simulink model "hop_2D_sim"  (R2022b)
settings: Solver=FixedStepAuto  StartTime=0.0  StopTime=0.5  FixedStep=10e-4  RelTol=1e-3
values from neighbouring files (symbols this model uses):
  bl = 0.1    [twoD.m]
  g = 9.81    [twoD.m]
  k0 = 1000    [twoD.m]
  Kf = acker(Af,Bf,Poles)    [twoD.m]
  l0 = 0.3    [twoD.m]
  m = 0.5    [twoD.m]
  Nf = rscale(Gp,Kf)    [twoD.m]
undefined symbols (not defined in the file or in its folder): If, K, Kg, Ts
settings Model: Creator=phattanarat  LastModifiedBy=phattanarat

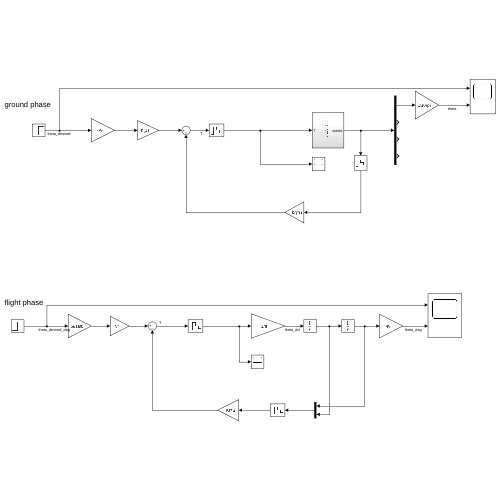
[thumbnail: Simulink's stored preview of the top-level diagram]
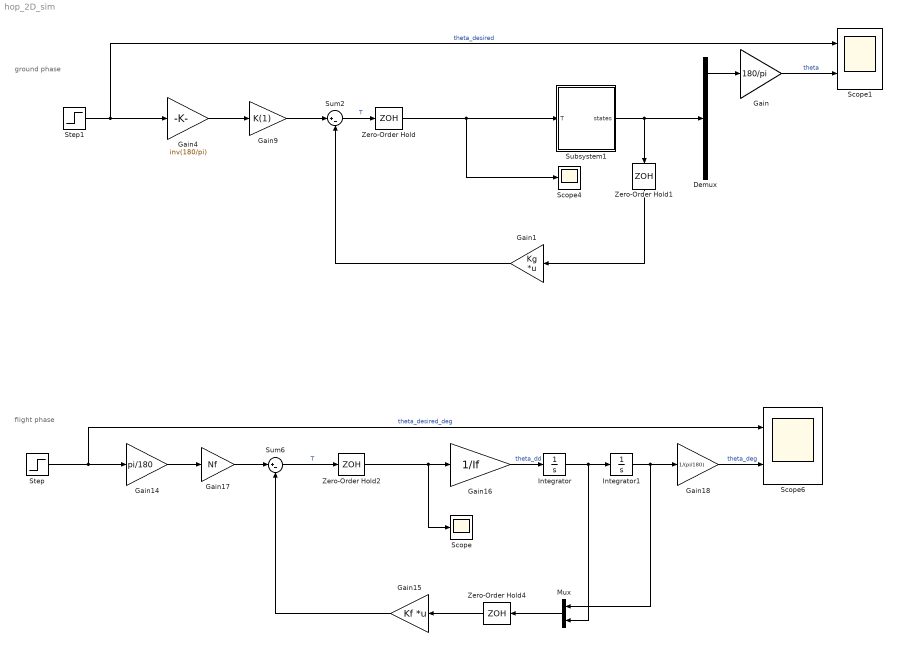
== system hop_2D_sim ==
  note: ground phase
  note: flight phase
  Demux : Demux
  Gain : Gain  Gain=180/pi
  Gain1 : Gain  Gain=Kg  Multiplication=Matrix(K*u)
  Gain14 : Gain  Gain=pi/180
  Gain15 : Gain  Gain=Kf  Multiplication=Matrix(K*u)
  Gain16 : Gain  Gain=1/If
  Gain17 : Gain  Gain=Nf
  Gain18 : Gain  Gain=1/(pi/180)
  Gain4 : Gain  Gain=inv(180/pi)
  Gain9 : Gain  Gain=K(1)
  Integrator : Integrator
  Integrator1 : Integrator  InitialCondition=deg2rad(95)
  Mux : Mux  Inputs=2
  Scope : Scope
  Scope1 : Scope  NumInputPorts=2
  Scope4 : Scope
  Scope6 : Scope  NumInputPorts=2
  Step : Step  Time=0  After=90  SampleTime=0
  Step1 : Step  Time=0  After=95  SampleTime=0
  Subsystem1 : Subsystem
  Sum2 : Sum  Inputs=|+-
  Sum6 : Sum  Inputs=|+-
  Zero-Order Hold{,1..2,4} (4 alike) : ZeroOrderHold  SampleTime=Ts
  wires:
  Gain9/1 -> Sum2/1
  Gain4/1 -> Gain9/1
  Sum2/1 -> Zero-Order Hold/1  "T"
  Step1/1 -> Scope1/1, Gain4/1  "theta_desired"
  Gain1/1 -> Sum2/2
  Gain14/1 -> Gain17/1
  Sum6/1 -> Zero-Order Hold2/1  "T"
  Gain16/1 -> Integrator/1  "theta_dd"
  Integrator1/1 -> Gain18/1, Mux/1
  Mux/1 -> Zero-Order Hold4/1
  Gain17/1 -> Sum6/1
  Gain18/1 -> Scope6/2  "theta_deg"
  Step/1 -> Scope6/1, Gain14/1  "theta_desired_deg"
  Subsystem1/1(states) -> Zero-Order Hold1/1, Demux/1
  Zero-Order Hold1/1 -> Gain1/1
  Demux/1 -> Gain/1
  Gain/1 -> Scope1/2  "theta"
  Integrator/1 -> Mux/2, Integrator1/1
  Zero-Order Hold4/1 -> Gain15/1
  Gain15/1 -> Sum6/2
  Zero-Order Hold/1 -> Scope4/1, Subsystem1/1(T)
  Zero-Order Hold2/1 -> Scope/1, Gain16/1

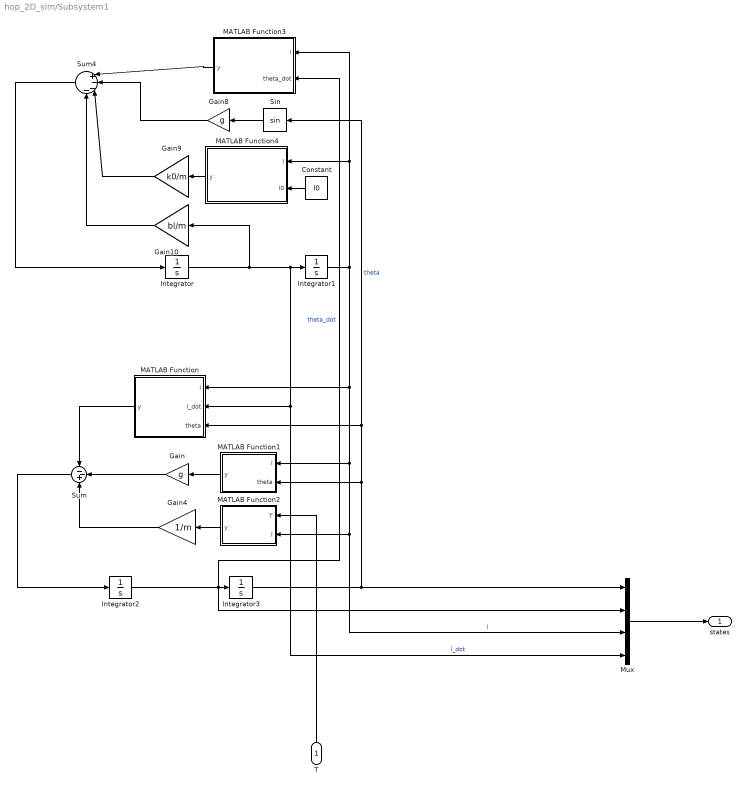
== system hop_2D_sim/Subsystem1 ==
  T : Inport
  Constant : Constant  Value=l0
  Gain : Gain  Gain=g
  Gain10 : Gain  Gain=bl/m
  Gain4 : Gain  Gain=1/m
  Gain8 : Gain  Gain=g
  Gain9 : Gain  Gain=k0/m
  Integrator : Integrator  InitialCondition=0.1
  Integrator1 : Integrator  InitialCondition=l0
  Integrator2 : Integrator
  Integrator3 : Integrator  InitialCondition=90*pi/180
  MATLAB Function : MATLAB Function  TreatAsAtomicUnit=on
  MATLAB Function1 : MATLAB Function  TreatAsAtomicUnit=on
  MATLAB Function2 : MATLAB Function  TreatAsAtomicUnit=on
  MATLAB Function3 : MATLAB Function  TreatAsAtomicUnit=on
  MATLAB Function4 : MATLAB Function  TreatAsAtomicUnit=on
  Mux : Mux
  Sin : Trigonometry
  Sum : Sum  Inputs=--+
  Sum4 : Sum  Inputs=|+---
  states : Outport
  wires:
  MATLAB Function4/1(y) -> Gain9/1
  MATLAB Function2/1(y) -> Gain4/1
  MATLAB Function1/1(y) -> Gain/1
  Integrator1/1 -> Mux/3, MATLAB Function2/2(l), MATLAB Function1/1(l), MATLAB Function/1(l), MATLAB Function4/1(l), MATLAB Function3/1(l)  "l"
  Integrator2/1 -> MATLAB Function3/2(theta_dot), Integrator3/1, Mux/2  "theta_dot"
  Sin/1 -> Gain8/1
  Integrator/1 -> Mux/4, MATLAB Function/2(l_dot), Integrator1/1, Gain10/1  "l_dot"
  Integrator3/1 -> MATLAB Function1/2(theta), MATLAB Function/3(theta), Sin/1, Mux/1  "theta"
  Constant/1 -> MATLAB Function4/2(l0)
  Gain/1 -> Sum/2
  Sum/1 -> Integrator2/1
  MATLAB Function/1(y) -> Sum/1
  Gain4/1 -> Sum/3
  T/1 -> MATLAB Function2/1(T)
  Sum4/1 -> Integrator/1
  MATLAB Function3/1(y) -> Sum4/1
  Gain8/1 -> Sum4/2
  Gain9/1 -> Sum4/3
  Gain10/1 -> Sum4/4
  Mux/1 -> states/1

== matlab function hop_2D_sim/Subsystem1/MATLAB Function1 ==
  data: l input; y output; theta input
function y = fcn(l,theta)

y = cos(theta)/l;

== matlab function hop_2D_sim/Subsystem1/MATLAB Function2 ==
  data: T input; l input; y output
function y = fcn(T,l)

y = T/l^2;

== matlab function hop_2D_sim/Subsystem1/MATLAB Function3 ==
  data: l input; y output; theta_dot input
function y = fcn(l,theta_dot)

y = l*theta_dot^2;

== matlab function hop_2D_sim/Subsystem1/MATLAB Function4 ==
  data: l input; y output; l0 input
function y = fcn(l,l0)

y = l-l0;

== matlab function hop_2D_sim/Subsystem1/MATLAB Function ==
  data: l input; l_dot input; y output; theta input
function y = fcn(l,l_dot,theta)

y = 2*l_dot*theta/l;
